simulink model "acc_decel_curv_plausibility"  (R2021a)
settings: Solver=VariableStepAuto  StartTime=0.0  StopTime=10.0  RelTol=1e-3
settings Model: Creator=uidk9388  LastModifiedBy=uidk9388

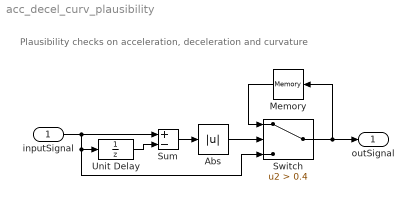
== system acc_decel_curv_plausibility ==
  note: Plausibility checks on acceleration, deceleration and curvature
  inputSignal : Inport
  Abs : Abs
  Memory : Memory
  Sum : Sum  Inputs=+-
  Switch : Switch  Criteria=u2 > Threshold  Threshold=0.4
  Unit Delay : UnitDelay  SampleTime=-1  HasFrameUpgradeWarning=on
  outSignal : Outport
  wires:
  Unit Delay/1 -> Sum/2
  Sum/1 -> Abs/1
  inputSignal/1 -> Switch/3, Unit Delay/1, Sum/1
  Abs/1 -> Switch/2
  Switch/1 -> Memory/1, outSignal/1
  Memory/1 -> Switch/1
